simulink model "ex_kalman11"  (R2017a)
settings: Solver=FixedStepDiscrete  StartTime=0.0  StopTime=309  RelTol=1e-3  EnableMultiTasking=on
InitFcn:
  | load position.mat;
  | [R,C]=size(position);
  | idx=(1:C)';
  | t=idx-1;
undefined symbols (not defined in the file or in its folder): position
settings Model: Creator=The MathWorks, Inc.  LastModifiedBy=The MathWorks, Inc.
settings DataIOCC: LimitDataPoints=on  SaveFormat=Array
settings OptimizationCC: ExpressionDepthLimit=2147483647  LifeSpan=inf
settings DebuggingCC: UnderspecifiedInitializationDetection=Classic  MergeDetectMultiDrivingBlocksExec=none  SolverPrmCheckMsg=warning  FcnCallInpInsideContextMsg=warning  StateNameClashWarn=warning  SFUnexpectedBacktrackingDiag=warning  SFNoUnconditionalDefaultTransitionDiag=warning  SFExecutionAtInitializationDiag=none
settings HardwareCC: ProdBitPerPointer=32  ProdBitPerSizeT=32  ProdBitPerPtrDiffT=32  ProdLargestAtomicFloat=None  ProdIntDivRoundTo=Undefined  ProdEndianess=Unspecified  ProdWordSize=32  ProdHWDeviceType=32-bit Generic
settings ModelReferenceCC: PropagateSignalLabelsOutOfModel=off
settings SFSimCC: SimParseCustomCode=off
settings GRTTargetCC: TargetLangStandard=C89/C90 (ANSI)  GeneratePreprocessorConditionals=Disable all  CombineOutputUpdateFcns=off  GRTInterface=on
settings ConfigComp: CovMetricSettings=dw  CovHtmlReporting=on  CovSaveCumulativeToWorkspaceVar=on  CovSaveSingleToWorkspaceVar=on  CovExternalEMLEnable=off

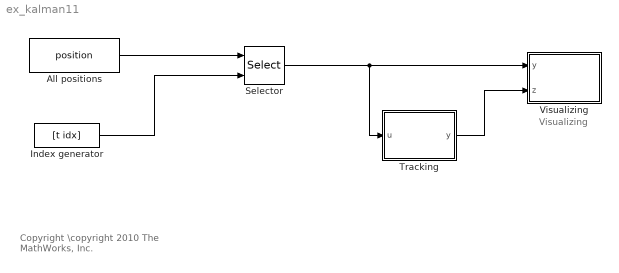
== system ex_kalman11 ==
  note: Visualizing
  note: Copyright \copyright 2010 The MathWorks, Inc.
  All positions : Constant  Value=position
  Index generator : FromWorkspace  VariableName=[t idx]  SampleTime=1  Interpolate=off  OutputAfterFinalValue=Holding final value
  Selector : Selector  NumberOfDimensions=2  InputPortWidth=2  IndexOptions=Select all,Index vector (port)  Indices=[1 3],2  OutputSizes=1,1
  Tracking : MATLAB Function  TreatAsAtomicUnit=on
  Visualizing : MATLAB Function  TreatAsAtomicUnit=on
  wires:
  All positions/1 -> Selector/1
  Index generator/1 -> Selector/2
  Selector/1 -> Tracking/1(u), Visualizing/1(y)
  Tracking/1(y) -> Visualizing/2(z)

== matlab function ex_kalman11/Visualizing ==
  data: y input; z input
function plot_me(y,z)
%#codegen

coder.extrinsic('figure','hold','plot_trajectory');
persistent h
if isempty(h)
  h=figure;
  hold;
end
plot_trajectory(y,z);
end

== matlab function ex_kalman11/Tracking ==
  data: u input; y output size=[2 1]
function y = kalman(u)
%#codegen

y = ex_kalman02(u);
